simulink model "MainSys"  (R2024b)
settings: Solver=VariableStepAuto  StartTime=0.0  StopTime=10.0  RelTol=1e-3
settings Model: Creator=mohammedazab  LastModifiedBy=mohammedazab

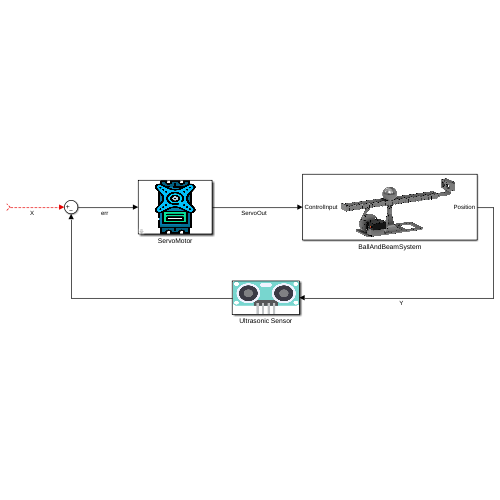
[thumbnail: Simulink's stored preview of the top-level diagram]
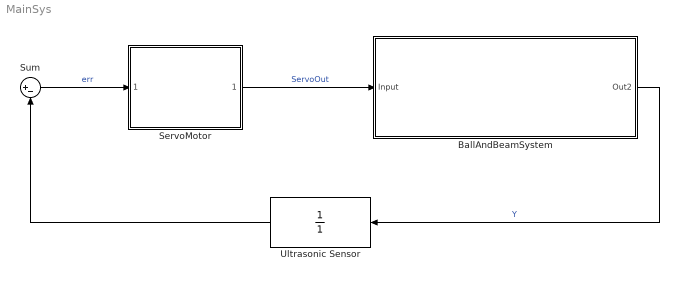
== system MainSys ==
  BallAndBeamSystem : Subsystem
      mask Display: image('BallbalanceSys.png');
  ServoMotor : Subsystem  ReferencedSubsystem=ServoMotor
  Sum : Sum  Inputs=|+-
  Ultrasonic Sensor : TransferFcn  Denominator=[1]
  wires:
  BallAndBeamSystem/1(Out2) -> Ultrasonic Sensor/1  "Y"
  Ultrasonic Sensor/1 -> Sum/2
  ? -> Sum/1  "X"
  Sum/1 -> ServoMotor/1  "err"
  ServoMotor/1 -> BallAndBeamSystem/1(Input)  "ServoOut"

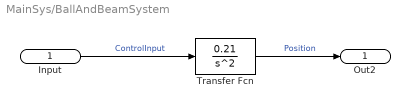
== system MainSys/BallAndBeamSystem ==
  Input : Inport
  Transfer Fcn : TransferFcn  Numerator=[0.21]  Denominator=[1 0 0]  ContinuousStateAttributes=position
  Out2 : Outport
  wires:
  Input/1 -> Transfer Fcn/1  "ControlInput"
  Transfer Fcn/1 -> Out2/1  "Position"
